simulink model "LugL7sStEnCtrl"  (R2024b)
settings: Solver=FixedStepDiscrete  StartTime=0.0  StopTime=10.0  FixedStep=0.01  RelTol=1e-3
undefined symbols (not defined in the file or in its folder): data, KeSMSw4SSecRwLtStLgrstOtwdInwdClosePos1_Val, KeSMSw4SSecRwLtStLgrstUpwdDnwdClosePos1_Val, KeSMSw4SSecRwLtStLgrstUpwdDnwdClosePos2_Val, SecRwLtStBkReclnEn_Clear, SecRwLtStBkReclnEn_Set, SecRwLtStFwdBkwdEn_Clear, SecRwLtStFwdBkwdEn_Set, SecRwLtStLgrstInwdOtwdEn_Clear, SecRwLtStLgrstInwdOtwdEn_Set, SecRwLtStLgrstUpwdDnwdEn_Clear, SecRwLtStLgrstUpwdDnwdEn_Set, SecRwRtStBkReclnEn_Clear, SecRwRtStBkReclnEn_Set, SecRwRtStFwdBkwdEn_Clear, SecRwRtStFwdBkwdEn_Set, SecRwRtStLgrstInwdOtwdEn_Clear, SecRwRtStLgrstInwdOtwdEn_Set, SecRwRtStLgrstUpwdDnwdEn_Clear, SecRwRtStLgrstUpwdDnwdEn_Set, ThdRwLtStBkReclnEn_Clear, ThdRwLtStBkReclnEn_Set, ThdRwLtStCshnFldEn_Clear, ThdRwLtStCshnFldEn_Set, ThdRwLtStFwdBkwdEn_Clear, ThdRwLtStFwdBkwdEn_Set, ZeroLEn_Clear, ZeroLEn_Set, ZeroREn_Clear, ZeroREn_Set
libraries: simulink x1
settings Model: Creator=sn2xws  LastModifiedBy=sn55gm
settings Model: ModifiedHistory=|
  | 2024.6.19 V1.0.0 模式流程V1.6
  | 2024.8.2 V3.0.0 模式流程V2.0
  | 2024.8.14 V3.0.1 修复三排前后可能无法到位的问题
  | 2024.8.23 V3.0.2 靠背折叠到位后，无法调用三排前后直接退出报失败的问题
  | 2024.8.26 V3.0.3 模式流程V2.4
  | 2024.8.30 V3.0.4 增加FirstTrig参数
  | 2024.9.3 V3.0.5 三排坐垫已折叠时，第一阶段不应该往前动三排前后位置
  | 2024.11.15 V3.0.6 增加二右到位置保持避免md8 md9同时调用时被清零
settings SolverCC: AlgebraicLoopSolver=TrustRegion
settings DataIOCC: SaveFormat=StructureWithTime  ReturnWorkspaceOutputs=off
settings OptimizationCC: DefaultParameterBehavior=Inlined  EnhancedBackFolding=on  PassReuseOutputArgsAs=Individual arguments  ZeroExternalMemoryAtStartup=off  ZeroInternalMemoryAtStartup=off  OptimizeBlockOrder=speed  DifferentSizesBufferReuse=on  OptimizationCustomize=off  EfficientTunableParamExpr=on
settings DebuggingCC: ParameterTunabilityLossMsg=error  UnconnectedInputMsg=warning  UnconnectedOutputMsg=warning  UnconnectedLineMsg=warning  ArithmeticOperatorsInVariantConditions=warning
settings ModelReferenceCC: EnableRefExpFcnMdlSchedulingChecks=on
settings SFSimCC: MATLABDynamicMemAlloc=off  CustomCodeUndefinedFunction=UseInterfaceOnly
settings RTWCC: Description=AUTOSAR  SystemTargetFile=autosar.tlc  GenCodeOnly=on  TemplateMakefile=ert_default_tmf  GenerateReport=on  IncludeHyperlinkInReport=on  LaunchReport=on  DataTypeReplacement=CDataTypesFixedWidth  GenerateTraceInfo=on  GenerateTraceReport=on  GenerateTraceReportSl=on  GenerateTraceReportSf=on  GenerateTraceReportEml=on  GPUComputeCapability=3.5
settings CodeAppCC: ForceParamTrailComments=on  IgnoreCustomStorageClasses=off  OperatorAnnotations=on  SimulinkDataObjDesc=on  SFDataObjDesc=on  InsertBlockDesc=on
settings STFCustomTargetCC: TargetLangStandard=C99 (ISO)  MultiwordLength=256  ParMdlRefBuildCompliant=on  CompOptLevelCompliant=on  IncludeMdlTerminateFcn=off  CombineOutputUpdateFcns=on  SuppressErrorStatus=on  ERTCustomFileBanners=on  SupportNonFinite=off  SupportComplex=off  SupportContinuousTime=off  SupportNonInlinedSFcns=off  RemoveResetFunc=on  MATLABClassNameForMDSCustomization=Simulink.SoftwareTarget.ERTCustomization  AutosarCompliant=on  UseToolchainInfoCompliant=on  LookupTableObjectStructAxisOrder=2,1,3,4,...  LUTObjectStructOrderEvenSpacing=Size,Table,Breakpoints  SystemTargetFile=autosar.tlc
settings ERTTargetCC: TargetLangStandard=C99 (ISO)  ConcurrentExecutionCompliant=off  IncludeMdlTerminateFcn=off  SuppressErrorStatus=on  SupportNonFinite=off  SupportComplex=off  ModelStepFunctionPrototypeControlCompliant=off  CPPClassGenCompliant=off  AutosarCompliant=on  LookupTableObjectStructAxisOrder=2,1,3,4,...  LUTObjectStructOrderEvenSpacing=Size,Table,Breakpoints  ERTCustomFileTemplate=example_file_process.tlc  ERTFilePackagingFormat=Compact  BooleanTrueId=TRUE  BooleanFalseId=FALSE  DynamicArrayContainerType=coder::array

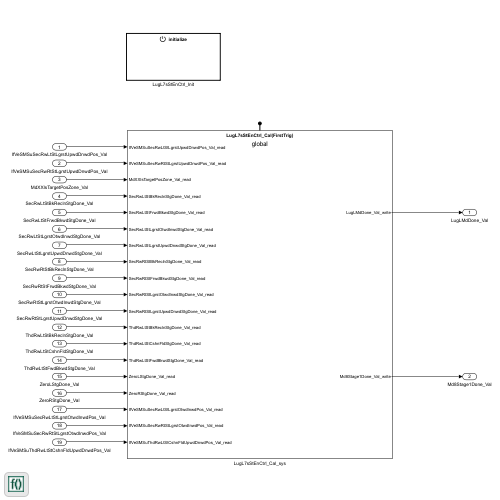
[thumbnail: Simulink's stored preview of the top-level diagram]
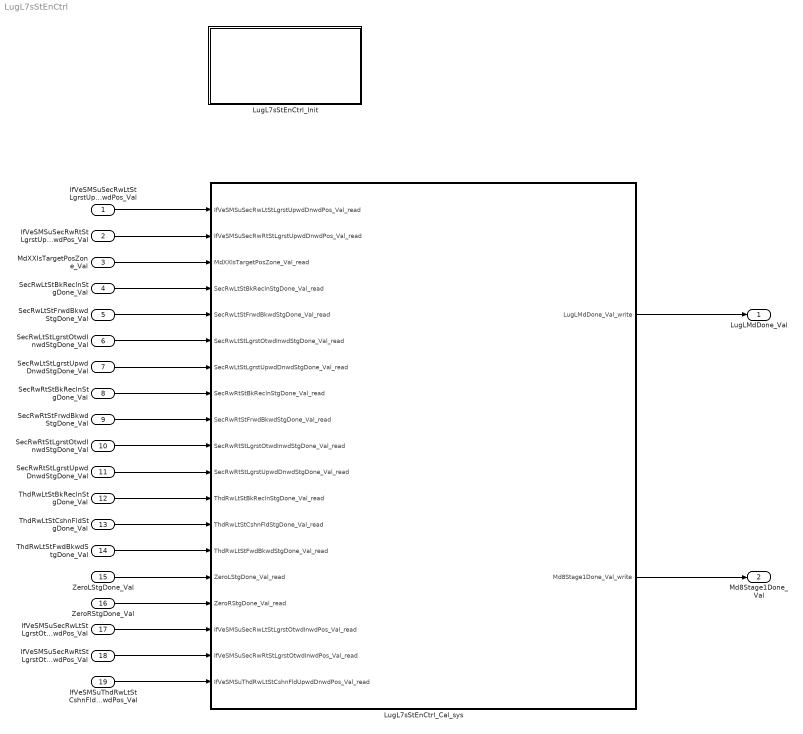
== system LugL7sStEnCtrl ==
  IfVeSMSuSecRwLtStLgrstUpwdDnwdPos_Val : Inport  OutDataTypeStr=uint16  PortDimensions=1
  IfVeSMSuSecRwRtStLgrstUpwdDnwdPos_Val : Inport  Port=2  OutDataTypeStr=uint16  PortDimensions=1
  MdXXIsTargetPosZone_Val : Inport  Port=3  OutDataTypeStr=uint32  PortDimensions=1
  SecRwLtStBkReclnStgDone_Val : Inport  Port=4  OutDataTypeStr=boolean  PortDimensions=1
  SecRwLtStFrwdBkwdStgDone_Val : Inport  Port=5  OutDataTypeStr=boolean  PortDimensions=1
  SecRwLtStLgrstOtwdInwdStgDone_Val : Inport  Port=6  OutDataTypeStr=boolean  PortDimensions=1
  SecRwLtStLgrstUpwdDnwdStgDone_Val : Inport  Port=7  OutDataTypeStr=boolean  PortDimensions=1
  SecRwRtStBkReclnStgDone_Val : Inport  Port=8  OutDataTypeStr=boolean  PortDimensions=1
  SecRwRtStFrwdBkwdStgDone_Val : Inport  Port=9  OutDataTypeStr=boolean  PortDimensions=1
  SecRwRtStLgrstOtwdInwdStgDone_Val : Inport  Port=10  OutDataTypeStr=boolean  PortDimensions=1
  SecRwRtStLgrstUpwdDnwdStgDone_Val : Inport  Port=11  OutDataTypeStr=boolean  PortDimensions=1
  ThdRwLtStBkReclnStgDone_Val : Inport  Port=12  OutDataTypeStr=boolean  PortDimensions=1
  ThdRwLtStCshnFldStgDone_Val : Inport  Port=13  OutDataTypeStr=boolean  PortDimensions=1
  ThdRwLtStFwdBkwdStgDone_Val : Inport  Port=14  OutDataTypeStr=boolean  PortDimensions=1
  ZeroLStgDone_Val : Inport  Port=15  OutDataTypeStr=boolean  PortDimensions=1
  ZeroRStgDone_Val : Inport  Port=16  OutDataTypeStr=boolean  PortDimensions=1
  IfVeSMSuSecRwLtStLgrstOtwdInwdPos_Val : Inport  Port=17  OutDataTypeStr=uint16  PortDimensions=1
  IfVeSMSuSecRwRtStLgrstOtwdInwdPos_Val : Inport  Port=18  OutDataTypeStr=uint16  PortDimensions=1
  IfVeSMSuThdRwLtStCshnFldUpwdDnwdPos_Val : Inport  Port=19  OutDataTypeStr=uint16  PortDimensions=1
  LugL7sStEnCtrl_Cal_sys : Subsystem
  LugL7sStEnCtrl_Init : Subsystem
  LugLMdDone_Val : Outport  OutDataTypeStr=uint8  PortDimensions=1  VectorParamsAs1DForOutWhenUnconnected=off
  Md8Stage1Done_Val : Outport  Port=2  OutDataTypeStr=boolean  PortDimensions=1  VectorParamsAs1DForOutWhenUnconnected=off
  wires:
  IfVeSMSuSecRwLtStLgrstUpwdDnwdPos_Val/1 -> LugL7sStEnCtrl_Cal_sys/1(IfVeSMSuSecRwLtStLgrstUpwdDnwdPos_Val_read)
  IfVeSMSuSecRwRtStLgrstUpwdDnwdPos_Val/1 -> LugL7sStEnCtrl_Cal_sys/2(IfVeSMSuSecRwRtStLgrstUpwdDnwdPos_Val_read)
  MdXXIsTargetPosZone_Val/1 -> LugL7sStEnCtrl_Cal_sys/3(MdXXIsTargetPosZone_Val_read)
  SecRwLtStBkReclnStgDone_Val/1 -> LugL7sStEnCtrl_Cal_sys/4(SecRwLtStBkReclnStgDone_Val_read)
  SecRwLtStFrwdBkwdStgDone_Val/1 -> LugL7sStEnCtrl_Cal_sys/5(SecRwLtStFrwdBkwdStgDone_Val_read)
  SecRwLtStLgrstOtwdInwdStgDone_Val/1 -> LugL7sStEnCtrl_Cal_sys/6(SecRwLtStLgrstOtwdInwdStgDone_Val_read)
  SecRwLtStLgrstUpwdDnwdStgDone_Val/1 -> LugL7sStEnCtrl_Cal_sys/7(SecRwLtStLgrstUpwdDnwdStgDone_Val_read)
  SecRwRtStBkReclnStgDone_Val/1 -> LugL7sStEnCtrl_Cal_sys/8(SecRwRtStBkReclnStgDone_Val_read)
  SecRwRtStFrwdBkwdStgDone_Val/1 -> LugL7sStEnCtrl_Cal_sys/9(SecRwRtStFrwdBkwdStgDone_Val_read)
  SecRwRtStLgrstOtwdInwdStgDone_Val/1 -> LugL7sStEnCtrl_Cal_sys/10(SecRwRtStLgrstOtwdInwdStgDone_Val_read)
  SecRwRtStLgrstUpwdDnwdStgDone_Val/1 -> LugL7sStEnCtrl_Cal_sys/11(SecRwRtStLgrstUpwdDnwdStgDone_Val_read)
  ThdRwLtStBkReclnStgDone_Val/1 -> LugL7sStEnCtrl_Cal_sys/12(ThdRwLtStBkReclnStgDone_Val_read)
  ThdRwLtStCshnFldStgDone_Val/1 -> LugL7sStEnCtrl_Cal_sys/13(ThdRwLtStCshnFldStgDone_Val_read)
  ThdRwLtStFwdBkwdStgDone_Val/1 -> LugL7sStEnCtrl_Cal_sys/14(ThdRwLtStFwdBkwdStgDone_Val_read)
  ZeroLStgDone_Val/1 -> LugL7sStEnCtrl_Cal_sys/15(ZeroLStgDone_Val_read)
  ZeroRStgDone_Val/1 -> LugL7sStEnCtrl_Cal_sys/16(ZeroRStgDone_Val_read)
  LugL7sStEnCtrl_Cal_sys/1(LugLMdDone_Val_write) -> LugLMdDone_Val/1
  IfVeSMSuSecRwLtStLgrstOtwdInwdPos_Val/1 -> LugL7sStEnCtrl_Cal_sys/17(IfVeSMSuSecRwLtStLgrstOtwdInwdPos_Val_read)
  IfVeSMSuSecRwRtStLgrstOtwdInwdPos_Val/1 -> LugL7sStEnCtrl_Cal_sys/18(IfVeSMSuSecRwRtStLgrstOtwdInwdPos_Val_read)
  IfVeSMSuThdRwLtStCshnFldUpwdDnwdPos_Val/1 -> LugL7sStEnCtrl_Cal_sys/19(IfVeSMSuThdRwLtStCshnFldUpwdDnwdPos_Val_read)
  LugL7sStEnCtrl_Cal_sys/2(Md8Stage1Done_Val_write) -> Md8Stage1Done_Val/1

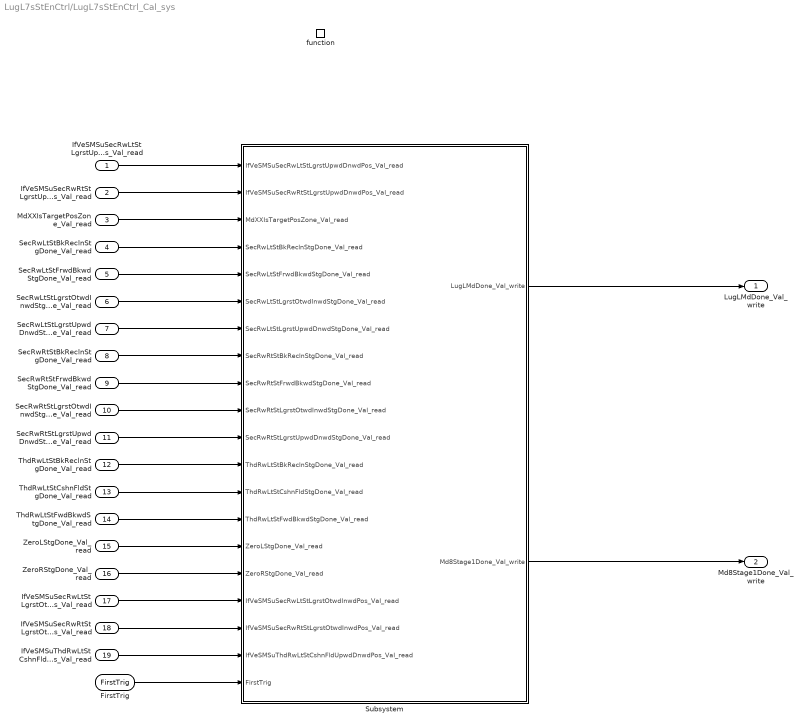
== system LugL7sStEnCtrl/LugL7sStEnCtrl_Cal_sys ==
  IfVeSMSuSecRwLtStLgrstUpwdDnwdPos_Val_read : Inport
  IfVeSMSuSecRwRtStLgrstUpwdDnwdPos_Val_read : Inport  Port=2
  MdXXIsTargetPosZone_Val_read : Inport  Port=3
  SecRwLtStBkReclnStgDone_Val_read : Inport  Port=4
  SecRwLtStFrwdBkwdStgDone_Val_read : Inport  Port=5
  SecRwLtStLgrstOtwdInwdStgDone_Val_read : Inport  Port=6
  SecRwLtStLgrstUpwdDnwdStgDone_Val_read : Inport  Port=7
  SecRwRtStBkReclnStgDone_Val_read : Inport  Port=8
  SecRwRtStFrwdBkwdStgDone_Val_read : Inport  Port=9
  SecRwRtStLgrstOtwdInwdStgDone_Val_read : Inport  Port=10
  SecRwRtStLgrstUpwdDnwdStgDone_Val_read : Inport  Port=11
  ThdRwLtStBkReclnStgDone_Val_read : Inport  Port=12
  ThdRwLtStCshnFldStgDone_Val_read : Inport  Port=13
  ThdRwLtStFwdBkwdStgDone_Val_read : Inport  Port=14
  ZeroLStgDone_Val_read : Inport  Port=15
  ZeroRStgDone_Val_read : Inport  Port=16
  IfVeSMSuSecRwLtStLgrstOtwdInwdPos_Val_read : Inport  Port=17
  IfVeSMSuSecRwRtStLgrstOtwdInwdPos_Val_read : Inport  Port=18
  IfVeSMSuThdRwLtStCshnFldUpwdDnwdPos_Val_read : Inport  Port=19
  function : TriggerPort  TriggerType=function-call  IsSimulinkFunction=on  FunctionName=LugL7sStEnCtrl_Cal  VariantControl=(inherit)
  Subsystem : Subsystem
  FirstTrig : ArgIn  OutDataTypeStr=boolean  ArgumentName=FirstTrig
  LugLMdDone_Val_write : Outport  VectorParamsAs1DForOutWhenUnconnected=off
      settings: EnsureOutportIsVirtual=on
  Md8Stage1Done_Val_write : Outport  Port=2  VectorParamsAs1DForOutWhenUnconnected=off
      settings: EnsureOutportIsVirtual=on
  wires:
  IfVeSMSuSecRwLtStLgrstUpwdDnwdPos_Val_read/1 -> Subsystem/1(IfVeSMSuSecRwLtStLgrstUpwdDnwdPos_Val_read)
  IfVeSMSuSecRwRtStLgrstUpwdDnwdPos_Val_read/1 -> Subsystem/2(IfVeSMSuSecRwRtStLgrstUpwdDnwdPos_Val_read)
  MdXXIsTargetPosZone_Val_read/1 -> Subsystem/3(MdXXIsTargetPosZone_Val_read)
  SecRwLtStBkReclnStgDone_Val_read/1 -> Subsystem/4(SecRwLtStBkReclnStgDone_Val_read)
  SecRwLtStFrwdBkwdStgDone_Val_read/1 -> Subsystem/5(SecRwLtStFrwdBkwdStgDone_Val_read)
  SecRwLtStLgrstOtwdInwdStgDone_Val_read/1 -> Subsystem/6(SecRwLtStLgrstOtwdInwdStgDone_Val_read)
  SecRwLtStLgrstUpwdDnwdStgDone_Val_read/1 -> Subsystem/7(SecRwLtStLgrstUpwdDnwdStgDone_Val_read)
  SecRwRtStBkReclnStgDone_Val_read/1 -> Subsystem/8(SecRwRtStBkReclnStgDone_Val_read)
  SecRwRtStFrwdBkwdStgDone_Val_read/1 -> Subsystem/9(SecRwRtStFrwdBkwdStgDone_Val_read)
  SecRwRtStLgrstOtwdInwdStgDone_Val_read/1 -> Subsystem/10(SecRwRtStLgrstOtwdInwdStgDone_Val_read)
  SecRwRtStLgrstUpwdDnwdStgDone_Val_read/1 -> Subsystem/11(SecRwRtStLgrstUpwdDnwdStgDone_Val_read)
  ThdRwLtStBkReclnStgDone_Val_read/1 -> Subsystem/12(ThdRwLtStBkReclnStgDone_Val_read)
  ThdRwLtStCshnFldStgDone_Val_read/1 -> Subsystem/13(ThdRwLtStCshnFldStgDone_Val_read)
  ThdRwLtStFwdBkwdStgDone_Val_read/1 -> Subsystem/14(ThdRwLtStFwdBkwdStgDone_Val_read)
  ZeroLStgDone_Val_read/1 -> Subsystem/15(ZeroLStgDone_Val_read)
  ZeroRStgDone_Val_read/1 -> Subsystem/16(ZeroRStgDone_Val_read)
  Subsystem/1(LugLMdDone_Val_write) -> LugLMdDone_Val_write/1
  IfVeSMSuSecRwLtStLgrstOtwdInwdPos_Val_read/1 -> Subsystem/17(IfVeSMSuSecRwLtStLgrstOtwdInwdPos_Val_read)
  IfVeSMSuSecRwRtStLgrstOtwdInwdPos_Val_read/1 -> Subsystem/18(IfVeSMSuSecRwRtStLgrstOtwdInwdPos_Val_read)
  IfVeSMSuThdRwLtStCshnFldUpwdDnwdPos_Val_read/1 -> Subsystem/19(IfVeSMSuThdRwLtStCshnFldUpwdDnwdPos_Val_read)
  Subsystem/2(Md8Stage1Done_Val_write) -> Md8Stage1Done_Val_write/1
  FirstTrig/1 -> Subsystem/20(FirstTrig)

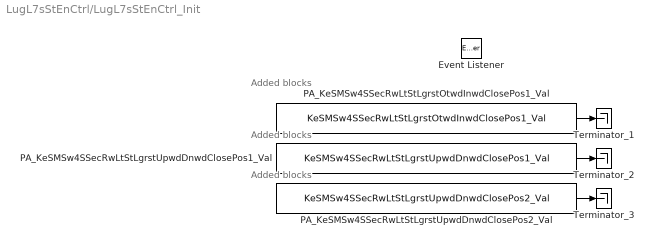
== system LugL7sStEnCtrl/LugL7sStEnCtrl_Init ==
  note: Added blocks
  note: Added blocks
  note: Added blocks
  Event Listener : EventListener  EventName=reset
  PA_KeSMSw4SSecRwLtStLgrstOtwdInwdClosePos1_Val : Constant  Value=KeSMSw4SSecRwLtStLgrstOtwdInwdClosePos1_Val
  PA_KeSMSw4SSecRwLtStLgrstUpwdDnwdClosePos1_Val : Constant  Value=KeSMSw4SSecRwLtStLgrstUpwdDnwdClosePos1_Val
  PA_KeSMSw4SSecRwLtStLgrstUpwdDnwdClosePos2_Val : Constant  Value=KeSMSw4SSecRwLtStLgrstUpwdDnwdClosePos2_Val
  Terminator_1 : Terminator
  Terminator_2 : Terminator
  Terminator_3 : Terminator
  wires:
  PA_KeSMSw4SSecRwLtStLgrstOtwdInwdClosePos1_Val/1 -> Terminator_1/1
  PA_KeSMSw4SSecRwLtStLgrstUpwdDnwdClosePos1_Val/1 -> Terminator_2/1
  PA_KeSMSw4SSecRwLtStLgrstUpwdDnwdClosePos2_Val/1 -> Terminator_3/1

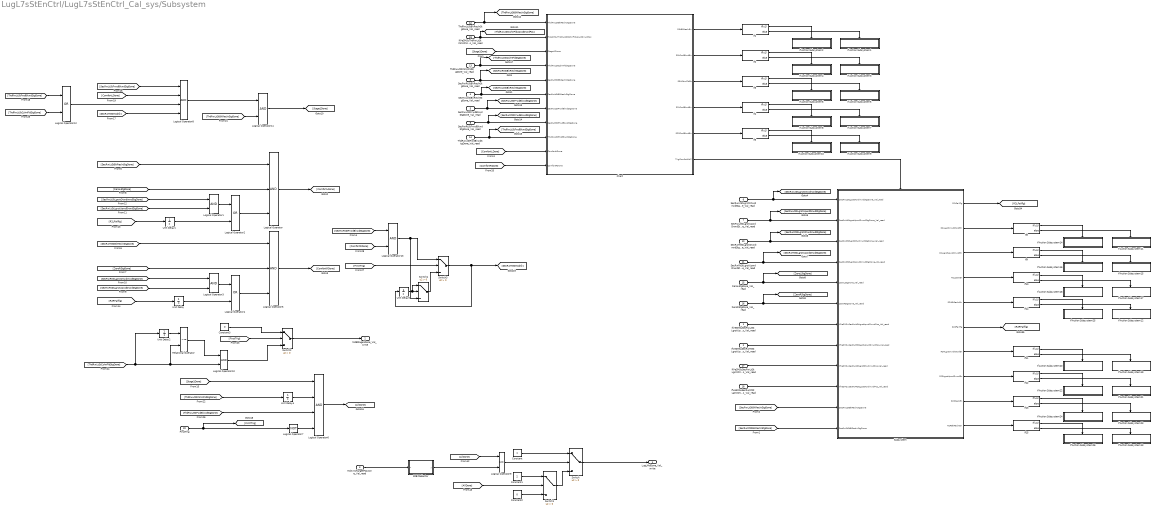
== system LugL7sStEnCtrl/LugL7sStEnCtrl_Cal_sys/Subsystem ==
  IfVeSMSuSecRwLtStLgrstUpwdDnwdPos_Val_read : Inport
  IfVeSMSuSecRwRtStLgrstUpwdDnwdPos_Val_read : Inport  Port=2
  MdXXIsTargetPosZone_Val_read : Inport  Port=3
  SecRwLtStBkReclnStgDone_Val_read : Inport  Port=4
  SecRwLtStFrwdBkwdStgDone_Val_read : Inport  Port=5
  SecRwLtStLgrstOtwdInwdStgDone_Val_read : Inport  Port=6
  SecRwLtStLgrstUpwdDnwdStgDone_Val_read : Inport  Port=7
  SecRwRtStBkReclnStgDone_Val_read : Inport  Port=8
  SecRwRtStFrwdBkwdStgDone_Val_read : Inport  Port=9
  SecRwRtStLgrstOtwdInwdStgDone_Val_read : Inport  Port=10
  SecRwRtStLgrstUpwdDnwdStgDone_Val_read : Inport  Port=11
  ThdRwLtStBkReclnStgDone_Val_read : Inport  Port=12
  ThdRwLtStCshnFldStgDone_Val_read : Inport  Port=13
  ThdRwLtStFwdBkwdStgDone_Val_read : Inport  Port=14
  ZeroLStgDone_Val_read : Inport  Port=15
  ZeroRStgDone_Val_read : Inport  Port=16
  IfVeSMSuSecRwLtStLgrstOtwdInwdPos_Val_read : Inport  Port=17
  IfVeSMSuSecRwRtStLgrstOtwdInwdPos_Val_read : Inport  Port=18
  IfVeSMSuThdRwLtStCshnFldUpwdDnwdPos_Val_read : Inport  Port=19
  FirstTrig : Inport  Port=20
  32BitSelector : Subsystem  mask(32 Bit Selector){BitNum=7}
      mask prompts: BitNum "Select Bit Number"
      mask help: Allows selection of a particular bit (0-31) out of a packed word up to 32 bits long. Output will be true if the bit number selected via the mask parameter is equal to one.
      mask TypeOptions BitNum: 0 | 1 | 2 | 3 | 4 | 5 | 6 | 7 | 8 | 9 | 10 | 11 | 12 | 13 | 14 | 15 | 16 | 17 | 18 | 19 | 20 | 21 | 22 | 23 | 24 | 25 | 26 | 27 | 28 | 29 | 30 | 31
      mask Display:
      | text(0.5, 0.8,'BIT','horizontalAlignment','center')
      | text(0.5, 0.5,'SELECTOR','horizontalAlignment','center')
      | text(0.5, 0.2,['-- Bit ',char(get_param(gcb,'BitNum')),' --'],'horizontalAlignment','center')
  Chart : Stateflow chart  TreatAsAtomicUnit=on
  Constant : Constant  OutDataTypeStr=uint8
  Constant1 : Constant  Value=2  OutDataTypeStr=uint8
  Constant2 : Constant  Value=0  OutDataTypeStr=uint8
  Constant3 : Constant  Value=0  OutDataTypeStr=boolean
  If Action Subsystem1 : Subsystem  TreatAsAtomicUnit=on
  If Action Subsystem10 : Subsystem  TreatAsAtomicUnit=on
  If Action Subsystem11 : Subsystem  TreatAsAtomicUnit=on
  If Action Subsystem12 : Subsystem  TreatAsAtomicUnit=on
  If Action Subsystem13 : Subsystem  TreatAsAtomicUnit=on
  If Action Subsystem14 : Subsystem  TreatAsAtomicUnit=on
  If Action Subsystem15 : Subsystem  TreatAsAtomicUnit=on
  If Action Subsystem16 : Subsystem  TreatAsAtomicUnit=on
  If Action Subsystem17 : Subsystem  TreatAsAtomicUnit=on
  If Action Subsystem18 : Subsystem  TreatAsAtomicUnit=on
  If Action Subsystem19 : Subsystem  TreatAsAtomicUnit=on
  If Action Subsystem2 : Subsystem  TreatAsAtomicUnit=on
  If Action Subsystem20 : Subsystem  TreatAsAtomicUnit=on
  If Action Subsystem21 : Subsystem  TreatAsAtomicUnit=on
  If Action Subsystem22 : Subsystem  TreatAsAtomicUnit=on
  If Action Subsystem23 : Subsystem  TreatAsAtomicUnit=on
  If Action Subsystem24 : Subsystem  TreatAsAtomicUnit=on
  If Action Subsystem25 : Subsystem  TreatAsAtomicUnit=on
  If Action Subsystem26 : Subsystem  TreatAsAtomicUnit=on
  If Action Subsystem3 : Subsystem  TreatAsAtomicUnit=on
  If Action Subsystem4 : Subsystem  TreatAsAtomicUnit=on
  If Action Subsystem5 : Subsystem  TreatAsAtomicUnit=on
  If Action Subsystem6 : Subsystem  TreatAsAtomicUnit=on
  If Action Subsystem7 : Subsystem  TreatAsAtomicUnit=on
  If Action Subsystem8 : Subsystem  TreatAsAtomicUnit=on
  If Action Subsystem9 : Subsystem  TreatAsAtomicUnit=on
  If{1..5,8..15} (13 alike) : If  IfExpression=u1
  Logical Operator : Logic  Inputs=3  AllPortsSameDT=off  OutDataTypeStr=boolean
  Logical Operator{1,3,9..11,13} (6 alike) : Logic  AllPortsSameDT=off  OutDataTypeStr=boolean
  Logical Operator12 : Logic  Operator=OR  AllPortsSameDT=off  OutDataTypeStr=boolean
  Logical Operator2 : Logic  Operator=OR  AllPortsSameDT=off  OutDataTypeStr=boolean
  Logical Operator4 : Logic  Operator=OR  AllPortsSameDT=off  OutDataTypeStr=boolean
  Logical Operator5 : Logic  Inputs=3  AllPortsSameDT=off  OutDataTypeStr=boolean
  Logical Operator6 : Logic  Inputs=4  AllPortsSameDT=off  OutDataTypeStr=boolean
  Logical Operator7 : Logic  Operator=NOT  Inputs=1  AllPortsSameDT=off  OutDataTypeStr=boolean
  Logical Operator8 : Logic  Inputs=4  AllPortsSameDT=off  OutDataTypeStr=boolean
  Relational Operator : RelationalOperator  Operator=~=  OutDataTypeStr=boolean  RndMeth=Simplest  InputSameDT=off
  Subsystem : Subsystem
  Switch{,1..4} (5 alike) : Switch  Criteria=u2 > Threshold  SaturateOnIntegerOverflow=off  InputSameDT=off
  Unit Delay{,1..4} (5 alike) : UnitDelay  SampleTime=-1  HasFrameUpgradeWarning=on
  LugLMdDone_Val_write : Outport  VectorParamsAs1DForOutWhenUnconnected=off
      settings: EnsureOutportIsVirtual=on
  Md8Stage1Done_Val_write : Outport  Port=2  VectorParamsAs1DForOutWhenUnconnected=off
      settings: EnsureOutportIsVirtual=on
  wires:
  IfVeSMSuSecRwLtStLgrstUpwdDnwdPos_Val_read/1 -> Subsystem/7(IfVeSMSuSecRwLtStLgrstUpwdDnwdPos_Val_read)
  IfVeSMSuSecRwRtStLgrstUpwdDnwdPos_Val_read/1 -> Subsystem/8(IfVeSMSuSecRwRtStLgrstUpwdDnwdPos_Val_read)
  SecRwLtStFrwdBkwdStgDone_Val_read/1 -> [SecRwLtStFrwdBkwdStgDone], Chart/7(SecRwLtStFrwdBkwdStgDone)
  SecRwLtStLgrstOtwdInwdStgDone_Val_read/1 -> [SecRwLtStLgrstOtwdInwdStgDone], Subsystem/1(SecRwLtStLgrstOtwdInwdStgDone_Val_read)
  SecRwRtStBkReclnStgDone_Val_read/1 -> [SecRwRtStBkReclnStgDone], Chart/5(SecRwRtStBkReclnStgDone)
  SecRwRtStFrwdBkwdStgDone_Val_read/1 -> [SecRwRtStFrwdBkwdStgDone], Chart/8(SecRwRtStFrwdBkwdStgDone)
  ThdRwLtStBkReclnStgDone_Val_read/1 -> [ThdRwLtStBkReclnStgDone], Chart/1(ThdRwLtStBkReclnStgDone)
  ThdRwLtStCshnFldStgDone_Val_read/1 -> [ThdRwLtStCshnFldStgDone], Chart/4(ThdRwLtStCshnFldStgDone)
  ZeroRStgDone_Val_read/1 -> [ZeroRStgDone], Subsystem/6(ZeroRStgDone_Val_read)
  Constant1/1 -> Switch1/1
  Switch/1 -> LugLMdDone_Val_write/1
  Logical Operator9/1 -> Switch/2
  Constant2/1 -> Switch1/3
  32BitSelector/1(y) -> Logical Operator9/2
  [AllDone] -> Logical Operator9/1
  Constant/1 -> Switch/1
  [AllDone] -> Switch1/2
  MdXXIsTargetPosZone_Val_read/1 -> 32BitSelector/1(x)
  Switch1/1 -> Switch/3
  IfVeSMSuThdRwLtStCshnFldUpwdDnwdPos_Val_read/1 -> [ThdRwLtStCshnFldUpwdDnwdPos], Chart/2(IfVeSMSuThdRwLtStCshnFldUpwdDnwdPos)
  [Stage1Done] -> Chart/3(Stage1Done)
  SecRwLtStBkReclnStgDone_Val_read/1 -> Chart/6(SecRwLtStBkReclnStgDone), [SecRwLtStBkReclnStgDone]
  Chart/6(TrigComfortMd()) -> Subsystem/Trigger
  IfVeSMSuSecRwRtStLgrstOtwdInwdPos_Val_read/1 -> Subsystem/10(IfVeSMSuSecRwRtStLgrstOtwdInwdPos_Val_read)
  IfVeSMSuSecRwLtStLgrstOtwdInwdPos_Val_read/1 -> Subsystem/9(IfVeSMSuSecRwLtStLgrstOtwdInwdPos_Val_read)
  SecRwRtStLgrstUpwdDnwdStgDone_Val_read/1 -> [SecRwRtStLgrstUpwdDnwdStgDone], Subsystem/4(SecRwRtStLgrstUpwdDnwdStgDone_Val_read)
  SecRwRtStLgrstOtwdInwdStgDone_Val_read/1 -> [SecRwRtStLgrstOtwdInwdStgDone], Subsystem/3(SecRwRtStLgrstOtwdInwdStgDone_Val_read)
  SecRwLtStLgrstUpwdDnwdStgDone_Val_read/1 -> [SecRwLtStLgrstUpwdDnwdStgDone], Subsystem/2(SecRwLtStLgrstUpwdDnwdStgDone_Val_read)
  [SecRwRtStBkReclnStgDone] -> Subsystem/12(SecRwRtStBkReclnStgDone)
  [SecRwLtStBkReclnStgDone] -> Subsystem/11(SecRwLtStBkReclnStgDone)
  ThdRwLtStFwdBkwdStgDone_Val_read/1 -> [ThdRwLtStFwdBkwdStgDone], Chart/9(ThdRwLtStFwdBkwdStgDone)
  Subsystem/6(R2RFailflg) -> [R2RFailflg]
  If13/1 -> If Action Subsystem24/Action
  If10/1 -> If Action Subsystem18/Action
  Subsystem/1(R2LFailflg) -> [R2LFailflg]
  Subsystem/7(R2RLgrstInwdOtwdEn) -> If11/1
  If11/2 -> If Action Subsystem19/Action
  If9/2 -> If Action Subsystem15/Action
  If14/1 -> If Action Subsystem25/Action
  If12/1 -> If Action Subsystem22/Action
  If13/2 -> If Action Subsystem23/Action
  Subsystem/4(R2LZeroEn) -> If10/1
  If10/2 -> If Action Subsystem17/Action
  If11/1 -> If Action Subsystem20/Action
  Subsystem/3(R2LLgrstUpwdDnwdEn) -> If9/1
  Subsystem/2(R2LLgrstInwdOtwdEn) -> If8/1
  If8/2 -> If Action Subsystem11/Action
  Subsystem/8(R2RLgrstUpwdDnwdEn) -> If12/1
  If12/2 -> If Action Subsystem21/Action
  Subsystem/5(R2LBkReclnEn) -> If14/1
  Subsystem/10(R2RBkReclnEn) -> If15/1
  If8/1 -> If Action Subsystem14/Action
  Subsystem/9(R2RZeroEn) -> If13/1
  If9/1 -> If Action Subsystem16/Action
  If15/1 -> If Action Subsystem26/Action
  If1/1 -> If Action Subsystem2/Action
  If1/2 -> If Action Subsystem1/Action
  Chart/1(R3LBkReclnEn) -> If1/1
  Chart/2(R3LFwdBkwdEn) -> If2/1
  If2/2 -> If Action Subsystem3/Action
  If2/1 -> If Action Subsystem4/Action
  If3/1 -> If Action Subsystem6/Action
  If3/2 -> If Action Subsystem5/Action
  Chart/3(R3LCshnFldEn) -> If3/1
  Chart/4(R2LFwdBkwdEn) -> If4/1
  If4/2 -> If Action Subsystem7/Action
  If4/1 -> If Action Subsystem8/Action
  If5/1 -> If Action Subsystem10/Action
  If5/2 -> If Action Subsystem9/Action
  Chart/5(R2RFwdBkwdEn) -> If5/1
  [ComfortLDone] -> Chart/10(ComfortLDone)
  [ComfortRDone] -> Chart/11(ComfortRDone)
  ZeroLStgDone_Val_read/1 -> [ZeroLStgDone], Subsystem/5(ZeroLStgDone_Val_read)
  [SecRwLtStLgrstOtwdInwdStgDone] -> Logical Operator1/1
  [SecRwLtStLgrstUpwdDnwdStgDone] -> Logical Operator1/2
  Logical Operator1/1 -> Logical Operator2/1
  [R2LFailflg] -> Unit Delay1/1
  [R2RFailflg] -> Unit Delay/1
  Logical Operator3/1 -> Logical Operator4/1
  [SecRwRtStLgrstUpwdDnwdStgDone] -> Logical Operator3/2
  [SecRwRtStLgrstOtwdInwdStgDone] -> Logical Operator3/1
  Logical Operator2/1 -> Logical Operator/3
  [ZeroLStgDone] -> Logical Operator/2
  [SecRwLtStBkReclnStgDone] -> Logical Operator/1
  Logical Operator4/1 -> Logical Operator5/3
  [ZeroRStgDone] -> Logical Operator5/2
  [SecRwRtStBkReclnStgDone] -> Logical Operator5/1
  Logical Operator/1 -> [ComfortLDone]
  Logical Operator5/1 -> [ComfortRDone]
  Logical Operator8/1 -> Logical Operator11/1
  [SecRwLtStFrwdBkwdStgDone] -> Logical Operator8/1
  If14/2 -> If Action Subsystem12/Action
  If15/2 -> If Action Subsystem13/Action
  Unit Delay/1 -> Logical Operator4/2
  Unit Delay1/1 -> Logical Operator2/2
  Logical Operator6/1 -> [AllDone]
  Switch2/1 -> Md8Stage1Done_Val_write/1
  [ThdRwLtStFwdBkwdStgDone] -> Logical Operator6/3
  [Stage1Done] -> Logical Operator6/1
  [ThdRwLtStCshnFldStgDone] -> Unit Delay4/1
  Logical Operator11/1 -> [Stage1Done]
  [ThdRwLtStBkReclnStgDone] -> Logical Operator11/2
  Unit Delay4/1 -> Logical Operator6/2
  Logical Operator7/1 -> Logical Operator6/4
  FirstTrig/1 -> [FirstTrig], Logical Operator7/1
  [FirstTrig] -> Switch2/2
  Constant3/1 -> Switch2/1
  Logical Operator10/1 -> Switch2/3
  Relational Operator/1 -> Logical Operator10/1
  [ThdRwLtStCshnFldStgDone] -> Unit Delay2/1, Relational Operator/2, Logical Operator10/2
  Unit Delay2/1 -> Relational Operator/1
  Logical Operator12/1 -> Logical Operator8/3
  [ThdRwLtStFwdBkwdStgDone] -> Logical Operator12/1
  [ThdRwLtStCshnFldStgDone] -> Logical Operator12/2
  [FirstTrig] -> Switch3/2
  Switch3/1 -> Unit Delay3/1, [SecRwRtStModify]
  [SecRwRtStFrwdBkwdStgDone] -> Logical Operator13/1
  [ComfortRDone] -> Logical Operator13/2
  Logical Operator13/1 -> Switch4/3, Switch3/1
  Unit Delay3/1 -> Switch4/1, Switch4/2
  Switch4/1 -> Switch3/3
  [ComfortLDone] -> Logical Operator8/2
  [SecRwRtStModify] -> Logical Operator8/4

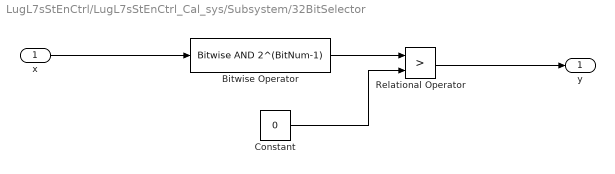
== system LugL7sStEnCtrl/LugL7sStEnCtrl_Cal_sys/Subsystem/32BitSelector ==
  x : Inport
  Bitwise Operator : simulink/Logic and Bit Operations/Bitwise Operator  logicop=AND  UseBitMask=on  BitMask=2^(BitNum-1)  BitMaskRealWorld=Stored Integer
  Constant : Constant  Value=0  OutDataTypeStr=uint32
  Relational Operator : RelationalOperator  Operator=>  OutDataTypeStr=boolean  RndMeth=Simplest  InputSameDT=off
  y : Outport  VectorParamsAs1DForOutWhenUnconnected=off
  wires:
  Relational Operator/1 -> y/1
  Constant/1 -> Relational Operator/2
  x/1 -> Bitwise Operator/1
  Bitwise Operator/1 -> Relational Operator/1

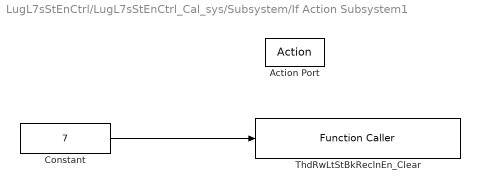
== system LugL7sStEnCtrl/LugL7sStEnCtrl_Cal_sys/Subsystem/If Action Subsystem1 ==
  Action Port : ActionPort  ActionPortLabel=else
  Constant : Constant  Value=7  OutDataTypeStr=uint8
  ThdRwLtStBkReclnEn_Clear : FunctionCaller  FunctionPrototype=ThdRwLtStBkReclnEn_Clear(data)  InputArgumentSpecifications=uint8(1)  OutputArgumentSpecifications=<Enter example>
  wires:
  Constant/1 -> ThdRwLtStBkReclnEn_Clear/1

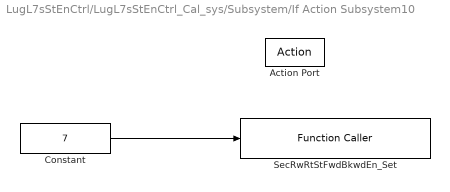
== system LugL7sStEnCtrl/LugL7sStEnCtrl_Cal_sys/Subsystem/If Action Subsystem10 ==
  Action Port : ActionPort  ActionPortLabel=if(u1)
  Constant : Constant  Value=7  OutDataTypeStr=uint8
  SecRwRtStFwdBkwdEn_Set : FunctionCaller  FunctionPrototype=SecRwRtStFwdBkwdEn_Set(data)  InputArgumentSpecifications=uint8(1)  OutputArgumentSpecifications=<Enter example>
  wires:
  Constant/1 -> SecRwRtStFwdBkwdEn_Set/1

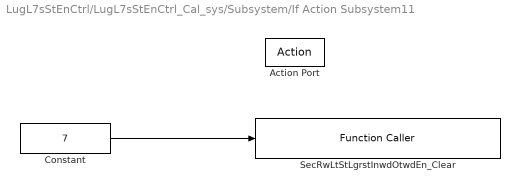
== system LugL7sStEnCtrl/LugL7sStEnCtrl_Cal_sys/Subsystem/If Action Subsystem11 ==
  Action Port : ActionPort  ActionPortLabel=else
  Constant : Constant  Value=7  OutDataTypeStr=uint8
  SecRwLtStLgrstInwdOtwdEn_Clear : FunctionCaller  FunctionPrototype=SecRwLtStLgrstInwdOtwdEn_Clear(data)  InputArgumentSpecifications=uint8(1)  OutputArgumentSpecifications=<Enter example>
  wires:
  Constant/1 -> SecRwLtStLgrstInwdOtwdEn_Clear/1

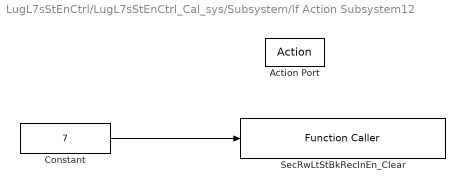
== system LugL7sStEnCtrl/LugL7sStEnCtrl_Cal_sys/Subsystem/If Action Subsystem12 ==
  Action Port : ActionPort  ActionPortLabel=else
  Constant : Constant  Value=7  OutDataTypeStr=uint8
  SecRwLtStBkReclnEn_Clear : FunctionCaller  FunctionPrototype=SecRwLtStBkReclnEn_Clear(data)  InputArgumentSpecifications=uint8(1)  OutputArgumentSpecifications=<Enter example>
  wires:
  Constant/1 -> SecRwLtStBkReclnEn_Clear/1

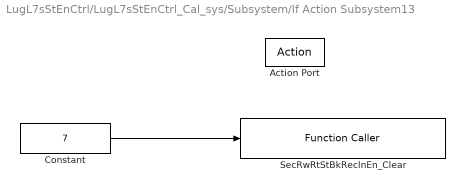
== system LugL7sStEnCtrl/LugL7sStEnCtrl_Cal_sys/Subsystem/If Action Subsystem13 ==
  Action Port : ActionPort  ActionPortLabel=else
  Constant : Constant  Value=7  OutDataTypeStr=uint8
  SecRwRtStBkReclnEn_Clear : FunctionCaller  FunctionPrototype=SecRwRtStBkReclnEn_Clear(data)  InputArgumentSpecifications=uint8(1)  OutputArgumentSpecifications=<Enter example>
  wires:
  Constant/1 -> SecRwRtStBkReclnEn_Clear/1

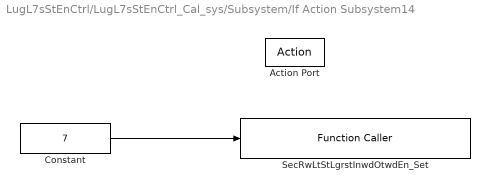
== system LugL7sStEnCtrl/LugL7sStEnCtrl_Cal_sys/Subsystem/If Action Subsystem14 ==
  Action Port : ActionPort  ActionPortLabel=if(u1)
  Constant : Constant  Value=7  OutDataTypeStr=uint8
  SecRwLtStLgrstInwdOtwdEn_Set : FunctionCaller  FunctionPrototype=SecRwLtStLgrstInwdOtwdEn_Set(data)  InputArgumentSpecifications=uint8(1)  OutputArgumentSpecifications=<Enter example>
  wires:
  Constant/1 -> SecRwLtStLgrstInwdOtwdEn_Set/1

== system LugL7sStEnCtrl/LugL7sStEnCtrl_Cal_sys/Subsystem/If Action Subsystem15 ==
  Action Port : ActionPort  ActionPortLabel=else
  Constant : Constant  Value=7  OutDataTypeStr=uint8
  SecRwLtStLgrstUpwdDnwdEn_Clear : FunctionCaller  FunctionPrototype=SecRwLtStLgrstUpwdDnwdEn_Clear(data)  InputArgumentSpecifications=uint8(1)  OutputArgumentSpecifications=<Enter example>
  wires:
  Constant/1 -> SecRwLtStLgrstUpwdDnwdEn_Clear/1

== system LugL7sStEnCtrl/LugL7sStEnCtrl_Cal_sys/Subsystem/If Action Subsystem16 ==
  Action Port : ActionPort  ActionPortLabel=if(u1)
  Constant : Constant  Value=7  OutDataTypeStr=uint8
  SecRwLtStLgrstUpwdDnwdEn_Set : FunctionCaller  FunctionPrototype=SecRwLtStLgrstUpwdDnwdEn_Set(data)  InputArgumentSpecifications=uint8(1)  OutputArgumentSpecifications=<Enter example>
  wires:
  Constant/1 -> SecRwLtStLgrstUpwdDnwdEn_Set/1

== system LugL7sStEnCtrl/LugL7sStEnCtrl_Cal_sys/Subsystem/If Action Subsystem17 ==
  Action Port : ActionPort  ActionPortLabel=else
  Constant : Constant  Value=7  OutDataTypeStr=uint8
  ZeroLEn_Clear : FunctionCaller  FunctionPrototype=ZeroLEn_Clear(data)  InputArgumentSpecifications=uint8(1)  OutputArgumentSpecifications=<Enter example>
  wires:
  Constant/1 -> ZeroLEn_Clear/1

== system LugL7sStEnCtrl/LugL7sStEnCtrl_Cal_sys/Subsystem/If Action Subsystem18 ==
  Action Port : ActionPort  ActionPortLabel=if(u1)
  Constant : Constant  Value=7  OutDataTypeStr=uint8
  ZeroLEn_Set : FunctionCaller  FunctionPrototype=ZeroLEn_Set(data)  InputArgumentSpecifications=uint8(1)  OutputArgumentSpecifications=<Enter example>
  wires:
  Constant/1 -> ZeroLEn_Set/1

== system LugL7sStEnCtrl/LugL7sStEnCtrl_Cal_sys/Subsystem/If Action Subsystem19 ==
  Action Port : ActionPort  ActionPortLabel=else
  Constant : Constant  Value=7  OutDataTypeStr=uint8
  SecRwRtStLgrstInwdOtwdEn_Clear : FunctionCaller  FunctionPrototype=SecRwRtStLgrstInwdOtwdEn_Clear(data)  InputArgumentSpecifications=uint8(1)  OutputArgumentSpecifications=<Enter example>
  wires:
  Constant/1 -> SecRwRtStLgrstInwdOtwdEn_Clear/1

== system LugL7sStEnCtrl/LugL7sStEnCtrl_Cal_sys/Subsystem/If Action Subsystem2 ==
  Action Port : ActionPort  ActionPortLabel=if(u1)
  Constant : Constant  Value=7  OutDataTypeStr=uint8
  ThdRwLtStBkReclnEn_Set : FunctionCaller  FunctionPrototype=ThdRwLtStBkReclnEn_Set(data)  InputArgumentSpecifications=uint8(1)  OutputArgumentSpecifications=<Enter example>
  wires:
  Constant/1 -> ThdRwLtStBkReclnEn_Set/1

== system LugL7sStEnCtrl/LugL7sStEnCtrl_Cal_sys/Subsystem/If Action Subsystem20 ==
  Action Port : ActionPort  ActionPortLabel=if(u1)
  Constant : Constant  Value=7  OutDataTypeStr=uint8
  SecRwRtStLgrstInwdOtwdEn_Set : FunctionCaller  FunctionPrototype=SecRwRtStLgrstInwdOtwdEn_Set(data)  InputArgumentSpecifications=uint8(1)  OutputArgumentSpecifications=<Enter example>
  wires:
  Constant/1 -> SecRwRtStLgrstInwdOtwdEn_Set/1

== system LugL7sStEnCtrl/LugL7sStEnCtrl_Cal_sys/Subsystem/If Action Subsystem21 ==
  Action Port : ActionPort  ActionPortLabel=else
  Constant : Constant  Value=7  OutDataTypeStr=uint8
  SecRwRtStLgrstUpwdDnwdEn_Clear : FunctionCaller  FunctionPrototype=SecRwRtStLgrstUpwdDnwdEn_Clear(data)  InputArgumentSpecifications=uint8(1)  OutputArgumentSpecifications=<Enter example>
  wires:
  Constant/1 -> SecRwRtStLgrstUpwdDnwdEn_Clear/1

== system LugL7sStEnCtrl/LugL7sStEnCtrl_Cal_sys/Subsystem/If Action Subsystem22 ==
  Action Port : ActionPort  ActionPortLabel=if(u1)
  Constant : Constant  Value=7  OutDataTypeStr=uint8
  SecRwRtStLgrstUpwdDnwdEn_Set : FunctionCaller  FunctionPrototype=SecRwRtStLgrstUpwdDnwdEn_Set(data)  InputArgumentSpecifications=uint8(1)  OutputArgumentSpecifications=<Enter example>
  wires:
  Constant/1 -> SecRwRtStLgrstUpwdDnwdEn_Set/1

== system LugL7sStEnCtrl/LugL7sStEnCtrl_Cal_sys/Subsystem/If Action Subsystem23 ==
  Action Port : ActionPort  ActionPortLabel=else
  Constant : Constant  Value=7  OutDataTypeStr=uint8
  ZeroREn_Clear : FunctionCaller  FunctionPrototype=ZeroREn_Clear(data)  InputArgumentSpecifications=uint8(1)  OutputArgumentSpecifications=<Enter example>
  wires:
  Constant/1 -> ZeroREn_Clear/1

== system LugL7sStEnCtrl/LugL7sStEnCtrl_Cal_sys/Subsystem/If Action Subsystem24 ==
  Action Port : ActionPort  ActionPortLabel=if(u1)
  Constant : Constant  Value=7  OutDataTypeStr=uint8
  ZeroREn_Set : FunctionCaller  FunctionPrototype=ZeroREn_Set(data)  InputArgumentSpecifications=uint8(1)  OutputArgumentSpecifications=<Enter example>
  wires:
  Constant/1 -> ZeroREn_Set/1

== system LugL7sStEnCtrl/LugL7sStEnCtrl_Cal_sys/Subsystem/If Action Subsystem25 ==
  note: Delete block
  Action Port : ActionPort  ActionPortLabel=if(u1)
  Constant : Constant  Value=7  OutDataTypeStr=uint8
  SecRwLtStBkReclnEn_Set : FunctionCaller  FunctionPrototype=SecRwLtStBkReclnEn_Set(data)  InputArgumentSpecifications=uint8(1)  OutputArgumentSpecifications=<Enter example>
  wires:
  Constant/1 -> SecRwLtStBkReclnEn_Set/1

== system LugL7sStEnCtrl/LugL7sStEnCtrl_Cal_sys/Subsystem/If Action Subsystem26 ==
  note: Delete block
  Action Port : ActionPort  ActionPortLabel=if(u1)
  Constant : Constant  Value=7  OutDataTypeStr=uint8
  SecRwRtStBkReclnEn_Set : FunctionCaller  FunctionPrototype=SecRwRtStBkReclnEn_Set(data)  InputArgumentSpecifications=uint8(1)  OutputArgumentSpecifications=<Enter example>
  wires:
  Constant/1 -> SecRwRtStBkReclnEn_Set/1

== system LugL7sStEnCtrl/LugL7sStEnCtrl_Cal_sys/Subsystem/If Action Subsystem3 ==
  Action Port : ActionPort  ActionPortLabel=else
  Constant : Constant  Value=7  OutDataTypeStr=uint8
  ThdRwLtStFwdBkwdEn_Clear : FunctionCaller  FunctionPrototype=ThdRwLtStFwdBkwdEn_Clear(data)  InputArgumentSpecifications=uint8(1)  OutputArgumentSpecifications=<Enter example>
  wires:
  Constant/1 -> ThdRwLtStFwdBkwdEn_Clear/1

== system LugL7sStEnCtrl/LugL7sStEnCtrl_Cal_sys/Subsystem/If Action Subsystem4 ==
  Action Port : ActionPort  ActionPortLabel=if(u1)
  Constant : Constant  Value=7  OutDataTypeStr=uint8
  ThdRwLtStFwdBkwdEn_Set : FunctionCaller  FunctionPrototype=ThdRwLtStFwdBkwdEn_Set(data)  InputArgumentSpecifications=uint8(1)  OutputArgumentSpecifications=<Enter example>
  wires:
  Constant/1 -> ThdRwLtStFwdBkwdEn_Set/1

== system LugL7sStEnCtrl/LugL7sStEnCtrl_Cal_sys/Subsystem/If Action Subsystem5 ==
  Action Port : ActionPort  ActionPortLabel=else
  Constant : Constant  Value=7  OutDataTypeStr=uint8
  ThdRwLtStCshnFldEn_Clear : FunctionCaller  FunctionPrototype=ThdRwLtStCshnFldEn_Clear(data)  InputArgumentSpecifications=uint8(1)  OutputArgumentSpecifications=<Enter example>
  wires:
  Constant/1 -> ThdRwLtStCshnFldEn_Clear/1

== system LugL7sStEnCtrl/LugL7sStEnCtrl_Cal_sys/Subsystem/If Action Subsystem6 ==
  Action Port : ActionPort  ActionPortLabel=if(u1)
  Constant : Constant  Value=7  OutDataTypeStr=uint8
  ThdRwLtStCshnFldEn_Set : FunctionCaller  FunctionPrototype=ThdRwLtStCshnFldEn_Set(data)  InputArgumentSpecifications=uint8(1)  OutputArgumentSpecifications=<Enter example>
  wires:
  Constant/1 -> ThdRwLtStCshnFldEn_Set/1

== system LugL7sStEnCtrl/LugL7sStEnCtrl_Cal_sys/Subsystem/If Action Subsystem7 ==
  Action Port : ActionPort  ActionPortLabel=else
  Constant : Constant  Value=7  OutDataTypeStr=uint8
  SecRwLtStFwdBkwdEn_Clear : FunctionCaller  FunctionPrototype=SecRwLtStFwdBkwdEn_Clear(data)  InputArgumentSpecifications=uint8(1)  OutputArgumentSpecifications=<Enter example>
  wires:
  Constant/1 -> SecRwLtStFwdBkwdEn_Clear/1

== system LugL7sStEnCtrl/LugL7sStEnCtrl_Cal_sys/Subsystem/If Action Subsystem8 ==
  Action Port : ActionPort  ActionPortLabel=if(u1)
  Constant : Constant  Value=7  OutDataTypeStr=uint8
  SecRwLtStFwdBkwdEn_Set : FunctionCaller  FunctionPrototype=SecRwLtStFwdBkwdEn_Set(data)  InputArgumentSpecifications=uint8(1)  OutputArgumentSpecifications=<Enter example>
  wires:
  Constant/1 -> SecRwLtStFwdBkwdEn_Set/1

== system LugL7sStEnCtrl/LugL7sStEnCtrl_Cal_sys/Subsystem/If Action Subsystem9 ==
  Action Port : ActionPort  ActionPortLabel=else
  Constant : Constant  Value=7  OutDataTypeStr=uint8
  SecRwRtStFwdBkwdEn_Clear : FunctionCaller  FunctionPrototype=SecRwRtStFwdBkwdEn_Clear(data)  InputArgumentSpecifications=uint8(1)  OutputArgumentSpecifications=<Enter example>
  wires:
  Constant/1 -> SecRwRtStFwdBkwdEn_Clear/1

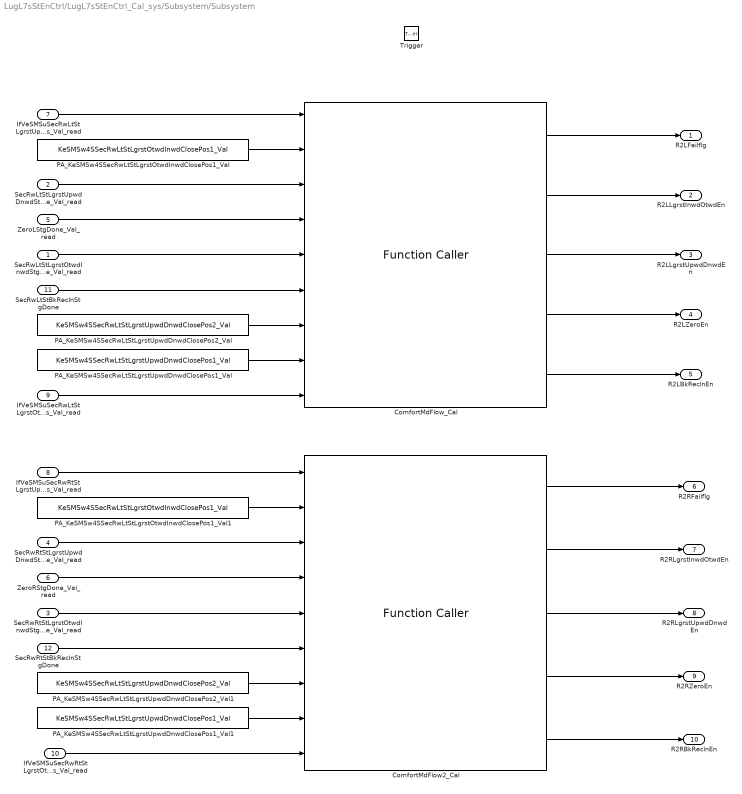
== system LugL7sStEnCtrl/LugL7sStEnCtrl_Cal_sys/Subsystem/Subsystem ==
  SecRwLtStLgrstOtwdInwdStgDone_Val_read : Inport
  SecRwLtStLgrstUpwdDnwdStgDone_Val_read : Inport  Port=2
  SecRwRtStLgrstOtwdInwdStgDone_Val_read : Inport  Port=3
  SecRwRtStLgrstUpwdDnwdStgDone_Val_read : Inport  Port=4
  ZeroLStgDone_Val_read : Inport  Port=5
  ZeroRStgDone_Val_read : Inport  Port=6
  IfVeSMSuSecRwLtStLgrstUpwdDnwdPos_Val_read : Inport  Port=7
  IfVeSMSuSecRwRtStLgrstUpwdDnwdPos_Val_read : Inport  Port=8
  IfVeSMSuSecRwLtStLgrstOtwdInwdPos_Val_read : Inport  Port=9
  IfVeSMSuSecRwRtStLgrstOtwdInwdPos_Val_read : Inport  Port=10
  SecRwLtStBkReclnStgDone : Inport  Port=11
  SecRwRtStBkReclnStgDone : Inport  Port=12
  Trigger : TriggerPort  TriggerType=function-call  VariantControl=Variant  PortDimensions=1
  ComfortMdFlow2_Cal : FunctionCaller  FunctionPrototype=[Failflg,LgrstInwdOtwdEn,LgrstUpwdDnwdEn,ZeroEn,BkReclnEn] = ComfortMdFlow2_Cal(LgrstUpwdDnwdPos,LgrstUpwdDnwdClosePos1,LgrstUpwdStgDone,ZeroStgDone,LgrstInwdStgDone,BkReclnStgDone,LgrstUpwdDnwdClosePos2,LgrstInwdOtwdClosePos1,LgrstInwdOtwdPos)  InputArgumentSpecifications=uint16(1), uint16(1), boolean(true), boolean(true), boolean(true), boolean(true), uint16(1), uint16(1), uint16(1)  OutputArgumentSpecifications=boolean(true), boolean(true), boolean(true), boolean(true), boolean(true)
  ComfortMdFlow_Cal : FunctionCaller  FunctionPrototype=[Failflg,LgrstInwdOtwdEn,LgrstUpwdDnwdEn,ZeroEn,BkReclnEn] = ComfortMdFlow_Cal(LgrstUpwdDnwdPos,LgrstUpwdDnwdClosePos1,LgrstUpwdStgDone,ZeroStgDone,LgrstInwdStgDone,BkReclnStgDone,LgrstUpwdDnwdClosePos2,LgrstInwdOtwdClosePos1,LgrstInwdOtwdPos)  InputArgumentSpecifications=uint16(1), uint16(1), boolean(true), boolean(true), boolean(true), boolean(true), uint16(1), uint16(1), uint16(1)  OutputArgumentSpecifications=boolean(true), boolean(true), boolean(true), boolean(true), boolean(true)
  PA_KeSMSw4SSecRwLtStLgrstOtwdInwdClosePos1_Val : Constant  Value=KeSMSw4SSecRwLtStLgrstOtwdInwdClosePos1_Val
  PA_KeSMSw4SSecRwLtStLgrstOtwdInwdClosePos1_Val1 : Constant  Value=KeSMSw4SSecRwLtStLgrstOtwdInwdClosePos1_Val
  PA_KeSMSw4SSecRwLtStLgrstUpwdDnwdClosePos1_Val : Constant  Value=KeSMSw4SSecRwLtStLgrstUpwdDnwdClosePos1_Val
  PA_KeSMSw4SSecRwLtStLgrstUpwdDnwdClosePos1_Val1 : Constant  Value=KeSMSw4SSecRwLtStLgrstUpwdDnwdClosePos1_Val
  PA_KeSMSw4SSecRwLtStLgrstUpwdDnwdClosePos2_Val : Constant  Value=KeSMSw4SSecRwLtStLgrstUpwdDnwdClosePos2_Val
  PA_KeSMSw4SSecRwLtStLgrstUpwdDnwdClosePos2_Val1 : Constant  Value=KeSMSw4SSecRwLtStLgrstUpwdDnwdClosePos2_Val
  R2LFailflg : Outport  VectorParamsAs1DForOutWhenUnconnected=off
  R2LLgrstInwdOtwdEn : Outport  Port=2  VectorParamsAs1DForOutWhenUnconnected=off
  R2LLgrstUpwdDnwdEn : Outport  Port=3  VectorParamsAs1DForOutWhenUnconnected=off
  R2LZeroEn : Outport  Port=4  VectorParamsAs1DForOutWhenUnconnected=off
  R2LBkReclnEn : Outport  Port=5  VectorParamsAs1DForOutWhenUnconnected=off
  R2RFailflg : Outport  Port=6  VectorParamsAs1DForOutWhenUnconnected=off
  R2RLgrstInwdOtwdEn : Outport  Port=7  VectorParamsAs1DForOutWhenUnconnected=off
  R2RLgrstUpwdDnwdEn : Outport  Port=8  VectorParamsAs1DForOutWhenUnconnected=off
  R2RZeroEn : Outport  Port=9  VectorParamsAs1DForOutWhenUnconnected=off
  R2RBkReclnEn : Outport  Port=10  VectorParamsAs1DForOutWhenUnconnected=off
  wires:
  PA_KeSMSw4SSecRwLtStLgrstUpwdDnwdClosePos1_Val1/1 -> ComfortMdFlow2_Cal/8
  PA_KeSMSw4SSecRwLtStLgrstOtwdInwdClosePos1_Val1/1 -> ComfortMdFlow2_Cal/2
  PA_KeSMSw4SSecRwLtStLgrstOtwdInwdClosePos1_Val/1 -> ComfortMdFlow_Cal/2
  SecRwRtStBkReclnStgDone/1 -> ComfortMdFlow2_Cal/6
  SecRwLtStBkReclnStgDone/1 -> ComfortMdFlow_Cal/6
  ZeroRStgDone_Val_read/1 -> ComfortMdFlow2_Cal/4
  PA_KeSMSw4SSecRwLtStLgrstUpwdDnwdClosePos2_Val/1 -> ComfortMdFlow_Cal/7
  IfVeSMSuSecRwLtStLgrstUpwdDnwdPos_Val_read/1 -> ComfortMdFlow_Cal/1
  IfVeSMSuSecRwRtStLgrstUpwdDnwdPos_Val_read/1 -> ComfortMdFlow2_Cal/1
  SecRwLtStLgrstUpwdDnwdStgDone_Val_read/1 -> ComfortMdFlow_Cal/3
  IfVeSMSuSecRwLtStLgrstOtwdInwdPos_Val_read/1 -> ComfortMdFlow_Cal/9
  SecRwLtStLgrstOtwdInwdStgDone_Val_read/1 -> ComfortMdFlow_Cal/5
  PA_KeSMSw4SSecRwLtStLgrstUpwdDnwdClosePos1_Val/1 -> ComfortMdFlow_Cal/8
  SecRwRtStLgrstOtwdInwdStgDone_Val_read/1 -> ComfortMdFlow2_Cal/5
  ZeroLStgDone_Val_read/1 -> ComfortMdFlow_Cal/4
  PA_KeSMSw4SSecRwLtStLgrstUpwdDnwdClosePos2_Val1/1 -> ComfortMdFlow2_Cal/7
  SecRwRtStLgrstUpwdDnwdStgDone_Val_read/1 -> ComfortMdFlow2_Cal/3
  IfVeSMSuSecRwRtStLgrstOtwdInwdPos_Val_read/1 -> ComfortMdFlow2_Cal/9
  ComfortMdFlow2_Cal/1 -> R2RFailflg/1
  ComfortMdFlow_Cal/2 -> R2LLgrstInwdOtwdEn/1
  ComfortMdFlow_Cal/4 -> R2LZeroEn/1
  ComfortMdFlow2_Cal/4 -> R2RZeroEn/1
  ComfortMdFlow2_Cal/5 -> R2RBkReclnEn/1
  ComfortMdFlow_Cal/5 -> R2LBkReclnEn/1
  ComfortMdFlow2_Cal/3 -> R2RLgrstUpwdDnwdEn/1
  ComfortMdFlow2_Cal/2 -> R2RLgrstInwdOtwdEn/1
  ComfortMdFlow_Cal/3 -> R2LLgrstUpwdDnwdEn/1
  ComfortMdFlow_Cal/1 -> R2LFailflg/1

== stateflow chart LugL7sStEnCtrl/LugL7sStEnCtrl_Cal_sys/Subsystem/Chart ==
  (default) -> (junction 1) : {
      | R3LBkReclnEn =0;
      | R3LCshnFldEn = 0;
      | R3LFwdBkwdEn =0;
      | R2LFwdBkwdEn=0;
      | R2RFwdBkwdEn = 0;
      | }
  (junction 1) -> (junction 3) [order 1] : [Stage1Done]
  (junction 3) -> (junction 208) [order 1] : [ThdRwLtStCshnFldStgDone]
  (junction 1) -> (junction 216) [order 2] : {
      | TrigComfortMd;
      | }
  (junction 3) -> (junction 7) [order 2] : {
      | R3LCshnFldEn = 1;
      | }
  (junction 208) -> (junction 289)
  (junction 231) -> (junction 252) [order 1] : [SecRwLtStFrwdBkwdStgDone]
  (junction 216) -> (junction 231) [order 1] : [ComfortLDone]
  (junction 252) -> (junction 256)
  (junction 216) -> (junction 235) [order 2]
  (junction 231) -> (junction 233) [order 2] : {
      | R2LFwdBkwdEn =1;
      | }
  (junction 256) -> (junction 233)
  (junction 233) -> (junction 235)
  (junction 235) -> (junction 248)
  (junction 248) -> (junction 250) [order 1] : [ComfortRDone]
  (junction 250) -> (junction 254) [order 1] : [SecRwRtStFrwdBkwdStgDone]
  (junction 248) -> (junction 262) [order 2]
  (junction 250) -> (junction 266) [order 2] : {
      | R2RFwdBkwdEn =1;
      | }
  (junction 254) -> (junction 259)
  (junction 266) -> (junction 262)
  (junction 259) -> (junction 266)
  (junction 262) -> (junction 221)
  (junction 221) -> (junction 223) [order 1] : [!ThdRwLtStBkReclnStgDone]
  (junction 221) -> (junction 227) [order 2]
  (junction 223) -> (junction 225) : {R3LBkReclnEn =1;}
  (junction 227) -> (junction 326) [order 1] : [ThdRwLtStFwdBkwdStgDone||ThdRwLtStCshnFldStgDone]
  (junction 227) -> (junction 244) [order 2] : {R3LFwdBkwdEn=1;}
  (junction 326) -> (junction 242)
  (junction 242) -> (junction 244)
  (junction 225) -> (junction 242)
  (junction 7) -> (junction 225)
  (junction 289) -> (junction 7)
  (junction 244) -> (junction 299)
  (junction 299) -> (junction 308) [order 1] : [ThdRwLtStCshnFldStgDone&&Stage1Done]
  (junction 308) -> (junction 333) [order 1] : [(ThdRwLtStFwdBkwdStgDone)]
  (junction 299) -> (junction 310) [order 2]
  (junction 308) -> (junction 314) [order 2] : {R3LFwdBkwdEn=1;
      | }
  (junction 333) -> (junction 335)
  (junction 314) -> (junction 310)
  (junction 335) -> (junction 314)
  (junction 310) -> (junction 320)
  data: ThdRwLtStBkReclnStgDone input; IfVeSMSuThdRwLtStCshnFldUpwdDnwdPos input; Stage1Done input boolean; R3LBkReclnEn output boolean; R3LFwdBkwdEn output boolean; R3LCshnFldEn output boolean; R2LFwdBkwdEn output boolean; ThdRwLtStCshnFldStgDone input; SecRwRtStBkReclnStgDone input; SecRwLtStBkReclnStgDone input; R2RFwdBkwdEn output boolean; SecRwLtStFrwdBkwdStgDone input; SecRwRtStFrwdBkwdStgDone input; ThdRwLtStFwdBkwdStgDone input; ComfortLDone input; ComfortRDone input
  events: TrigComfortMd output FUNCTION_CALL_EVENT
